simulink model "CSRT_Discreto"  (R2020b)
settings: Solver=FixedStepAuto  StartTime=0.0  StopTime=15  FixedStep=0.01  RelTol=1e-3
values from neighbouring files (symbols this model uses):
  A = [A11, A12; A21, A22]    [Exp2_CSRT.m]
  B = horzcat(Bu, Bd)    [Exp2_CSRT.m]
  C = [1, 0]    [Exp2_CSRT.m]
  Cas = 8.564    [Exp2_CSRT.m]
  D = [0, 0, 0, 0]    [Exp2_CSRT.m]
  Gdisc1 = c2d(Gss, 0.2, 'zoh')    [Exp2_CSRT.m]
  Gdisc2 = c2d(Gss, 0.5, 'zoh')    [Exp2_CSRT.m]
  Gdisc3 = c2d(Gss, 1.5, 'zoh')    [Exp2_CSRT.m]
settings Model: Creator=franc  LastModifiedBy=franc

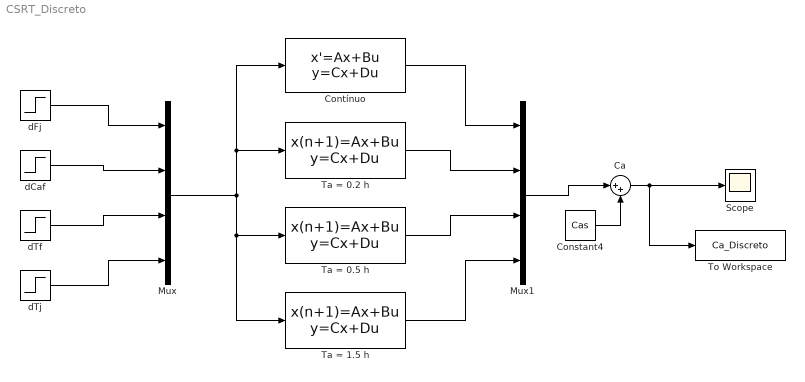
== system CSRT_Discreto ==
  "            Ca" : Sum  Inputs=|++
  Constant4 : Constant  Value=Cas
  Contínuo : StateSpace  A=A  B=B  C=C  D=D  InitialCondition=0
  Mux : Mux
  Mux1 : Mux
  Scope : Scope
  Ta = 0.2 h : DiscreteStateSpace  A=Gdisc1.A  B=Gdisc1.B  C=Gdisc1.C  D=Gdisc1.D  SampleTime=0.2
  Ta = 0.5 h : DiscreteStateSpace  A=Gdisc2.A  B=Gdisc2.B  C=Gdisc2.C  D=Gdisc2.D  SampleTime=0.5
  Ta = 1.5 h : DiscreteStateSpace  A=Gdisc3.A  B=Gdisc3.B  C=Gdisc3.C  D=Gdisc3.D  SampleTime=1.5
  To Workspace : ToWorkspace  VariableName=Ca_Discreto  SaveFormat=Timeseries  SampleTime=-1
  dCaf : Step  Time=0  After=0  SampleTime=0
  dFj : Step  Time=0  After=0.01  SampleTime=0
  dTf : Step  Time=0  After=0  SampleTime=0
  dTj : Step  Time=0  After=0  SampleTime=0
  wires:
  dFj/1 -> Mux/1
  dTf/1 -> Mux/3
  Mux1/1 -> "            Ca"/1
  "            Ca"/1 -> Scope/1, To Workspace/1
  Contínuo/1 -> Mux1/1
  Constant4/1 -> "            Ca"/2
  Ta = 1.5 h/1 -> Mux1/4
  Mux/1 -> Contínuo/1, Ta = 0.2 h/1, Ta = 0.5 h/1, Ta = 1.5 h/1
  dTj/1 -> Mux/4
  dCaf/1 -> Mux/2
  Ta = 0.5 h/1 -> Mux1/3
  Ta = 0.2 h/1 -> Mux1/2
